simulink library "Brakes_None"  (R2019a)
settings: Solver=VariableStepAuto  StartTime=0.0  StopTime=10.0  RelTol=1e-3
libraries: fl_lib x6
Description:
  | Component of Simscape Vehicle Templates Library
  | 
  | Copyright 2018-2020 The MathWorks, Inc.
settings Model: Creator=smiller  LastModifiedBy=smiller
settings DataIOCC: ReturnWorkspaceOutputs=off
settings DebuggingCC: ArithmeticOperatorsInVariantConditions=warning

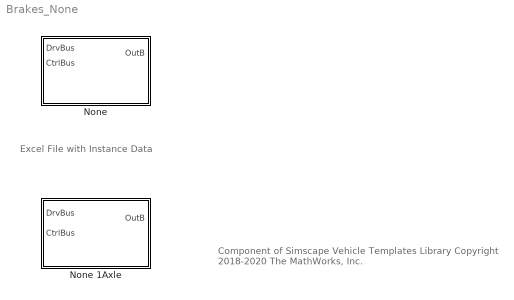
== system Brakes_None ==
  note: Excel File with Instance Data
  note: Component of Simscape Vehicle Templates Library
      | Copyright 2018-2020 The MathWorks, Inc.
  None : Subsystem  Tag=PublishSubsystem  VariantControl=Pedal  mask(Brake System, Pedal Input){}
  None 1Axle : Subsystem  Tag=PublishSubsystem  VariantControl=Pedal  mask(Brake System, Pedal Input){}

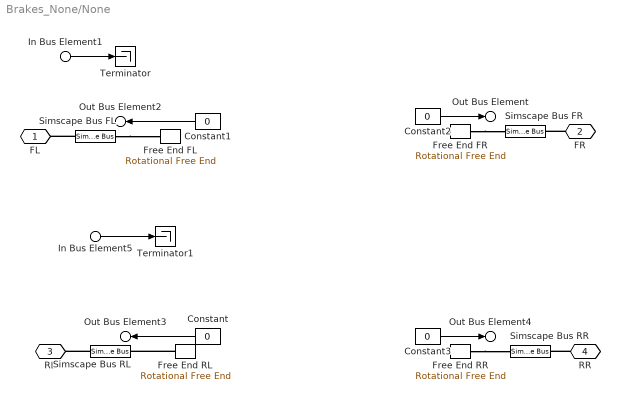
== system Brakes_None/None ==
  In Bus Element5 : Inport  PortName=DrvBus  Element=rBrakePedal
  In Bus Element1 : Inport  Port=2  PortName=CtrlBus
  Constant{,1..3} (4 alike) : Constant  Value=0
  Free End FL : fl_lib/Mechanical/Rotational Elements/Rotational Free End  w_specify=off  w_priority=None  w=0 rad/s  w_nominal_specify=off  w_nominal_unit=rad/s  w_nominal_value=1
      settings: SourceProductName=Simscape  SourceProductBaseCode=SS
  Free End FR : fl_lib/Mechanical/Rotational Elements/Rotational Free End  w_specify=off  w_priority=None  w=0 rad/s  w_nominal_specify=off  w_nominal_unit=rad/s  w_nominal_value=1
      settings: SourceProductName=Simscape  SourceProductBaseCode=SS
  Free End RL : fl_lib/Mechanical/Rotational Elements/Rotational Free End  w_specify=off  w_priority=None  w=0 rad/s  w_nominal_specify=off  w_nominal_unit=rad/s  w_nominal_value=1
      settings: SourceProductName=Simscape  SourceProductBaseCode=SS
  Free End RR : fl_lib/Mechanical/Rotational Elements/Rotational Free End  w_specify=off  w_priority=None  w=0 rad/s  w_nominal_specify=off  w_nominal_unit=rad/s  w_nominal_value=1
      settings: SourceProductName=Simscape  SourceProductBaseCode=SS
  Simscape Bus FL : SimscapeBus  HierarchyStrings=Axle1D
  Simscape Bus FR : SimscapeBus  HierarchyStrings=Axle1D
  Simscape Bus RL : SimscapeBus  HierarchyStrings=Axle1D
  Simscape Bus RR : SimscapeBus  HierarchyStrings=Axle1D
  Terminator : Terminator
  Terminator1 : Terminator
  FL : PMIOPort  Side=Left
  FR : PMIOPort  Port=2  Side=Right
  RL : PMIOPort  Port=3  Side=Left
  RR : PMIOPort  Port=4  Side=Right
  Out Bus Element2 : Outport  PortName=OutB  Element=MBrakeFL
  Out Bus Element : Outport  PortName=OutB  Element=MBrakeFR
  Out Bus Element3 : Outport  PortName=OutB  Element=MBrakeRL
  Out Bus Element4 : Outport  PortName=OutB  Element=MBrakeRR
  wires:
  Constant3/1 -> Out Bus Element4/1
  Constant/1 -> Out Bus Element3/1
  Constant2/1 -> Out Bus Element/1
  Constant1/1 -> Out Bus Element2/1
  In Bus Element1/1 -> Terminator/1
  In Bus Element5/1 -> Terminator1/1
  connections:
  Free End RR/LConn1 -- Simscape Bus RR/LConn1
  Free End RL/LConn1 -- Simscape Bus RL/LConn1
  Free End FR/LConn1 -- Simscape Bus FR/LConn1
  Simscape Bus FL/LConn1 -- Free End FL/LConn1
  Simscape Bus FL/RConn1 -- FL/RConn1
  Simscape Bus RL/RConn1 -- RL/RConn1
  RR/RConn1 -- Simscape Bus RR/RConn1
  FR/RConn1 -- Simscape Bus FR/RConn1

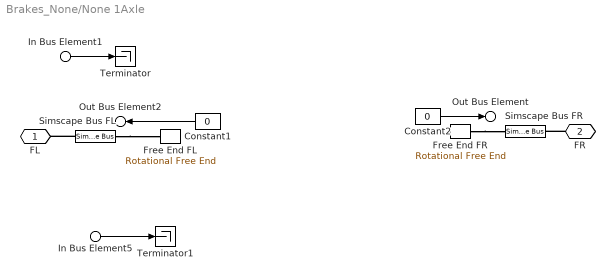
== system Brakes_None/None 1Axle ==
  In Bus Element5 : Inport  PortName=DrvBus  Element=rBrakePedal
  In Bus Element1 : Inport  Port=2  PortName=CtrlBus
  Constant1 : Constant  Value=0
  Constant2 : Constant  Value=0
  Free End FL : fl_lib/Mechanical/Rotational Elements/Rotational Free End  w_specify=off  w_priority=None  w=0 rad/s  w_nominal_specify=off  w_nominal_unit=rad/s  w_nominal_value=1
      settings: SourceProductName=Simscape  SourceProductBaseCode=SS
  Free End FR : fl_lib/Mechanical/Rotational Elements/Rotational Free End  w_specify=off  w_priority=None  w=0 rad/s  w_nominal_specify=off  w_nominal_unit=rad/s  w_nominal_value=1
      settings: SourceProductName=Simscape  SourceProductBaseCode=SS
  Simscape Bus FL : SimscapeBus  HierarchyStrings=Axle1D
  Simscape Bus FR : SimscapeBus  HierarchyStrings=Axle1D
  Terminator : Terminator
  Terminator1 : Terminator
  FL : PMIOPort  Side=Left
  FR : PMIOPort  Port=2  Side=Right
  Out Bus Element2 : Outport  PortName=OutB  Element=MBrakeFL
  Out Bus Element : Outport  PortName=OutB  Element=MBrakeFR
  wires:
  In Bus Element5/1 -> Terminator1/1
  In Bus Element1/1 -> Terminator/1
  Constant1/1 -> Out Bus Element2/1
  Constant2/1 -> Out Bus Element/1
  connections:
  FR/RConn1 -- Simscape Bus FR/RConn1
  Simscape Bus FL/RConn1 -- FL/RConn1
  Simscape Bus FL/LConn1 -- Free End FL/LConn1
  Free End FR/LConn1 -- Simscape Bus FR/LConn1
